simulink model "lab3_symulacja"  (R2022a)
settings: Solver=VariableStepAuto  StartTime=0.0  StopTime=30.0  RelTol=1e-3
values from neighbouring files (symbols this model uses):
  A = [0, 1, 0, 0 ... (first row only)    [lab3.m]
  B = [0; 1/M; 0; 1/M*L]    [lab3.m]
  C = eye(4)    [lab3.m]
  D = [0 ... (first row only)    [lab3.m]
  K = lqr(system, Q, R)    [lab3.m]
  x = [1 ... (first row only)    [lab3.m]
settings Model: Creator=rober  LastModifiedBy=rober

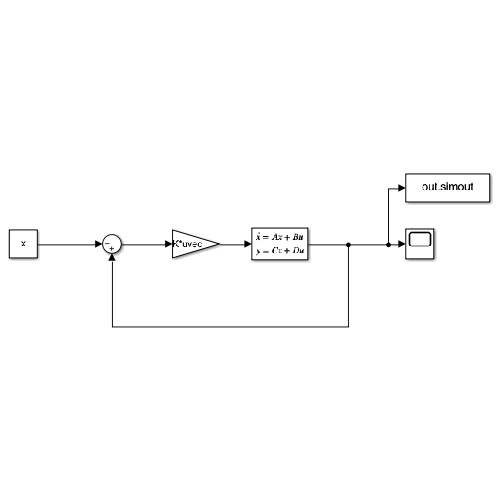
[thumbnail: Simulink's stored preview of the top-level diagram]
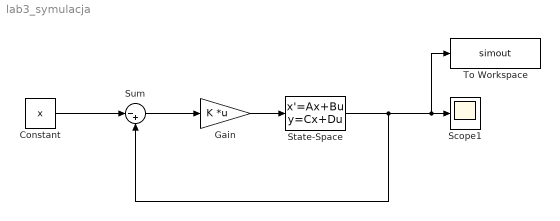
== system lab3_symulacja ==
  Constant : Constant  Value=x
  Gain : Gain  Gain=K  Multiplication=Matrix(K*u) (u vector)
  Scope1 : Scope
  State-Space : StateSpace  A=A  B=B  C=C  D=D  InitialCondition=0
  Sum : Sum  Inputs=|-+
  To Workspace : ToWorkspace  VariableName=simout  SampleTime=-1
  wires:
  Sum/1 -> Gain/1
  Constant/1 -> Sum/1
  Gain/1 -> State-Space/1
  State-Space/1 -> Sum/2, To Workspace/1, Scope1/1
